simulink library "Window_Optics"  (Simulink 8.2)
settings: Solver=ode45  StartTime=0.0  StopTime=10.0  RelTol=1e-3
settings Model: Creator=lena.frank  LastModifiedBy=drhf

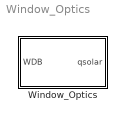
== system Window_Optics ==
  Window_Optics : Subsystem

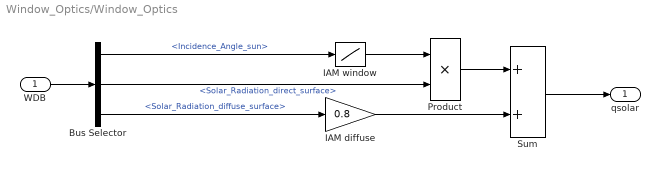
== system Window_Optics/Window_Optics ==
  WDB : Inport
  Bus Selector : BusSelector  OutputSignals=Incidence_Angle_sun,Solar_Radiation_direct_surface,Solar_Radiation_diffuse_surface
  IAM diffuse : Gain  Gain=0.8  SaturateOnIntegerOverflow=on  OutDataTypeStr=Inherit: Same as input  ParamDataTypeStr=Inherit: Same as input
  IAM window : Lookup  InputValues=[-10 0 50 70 80 90]  Table="[1.0 1.0  0.95  0.7  0.0  0.0]"  SaturateOnIntegerOverflow=on
  Product : Product
  Sum : Sum  SaturateOnIntegerOverflow=on  InputSameDT=on  OutDataTypeStr=Inherit: Same as first input
  qsolar : Outport
  wires:
  WDB/1 -> Bus Selector/1
  Bus Selector/2 -> Product/2  "<Solar_Radiation_direct_surface>"
  Bus Selector/1 -> IAM window/1  "<Incidence_Angle_sun>"
  Sum/1 -> qsolar/1
  Product/1 -> Sum/1
  IAM diffuse/1 -> Sum/2
  IAM window/1 -> Product/1
  Bus Selector/3 -> IAM diffuse/1  "<Solar_Radiation_diffuse_surface>"
